simulink library "filters"  (R2024b)
settings: Solver=VariableStepAuto  StartTime=0.0  StopTime=10.0  RelTol=1e-3
libraries: simulink x1
settings Model: Creator=upattacini  LastModifiedBy=upattacini

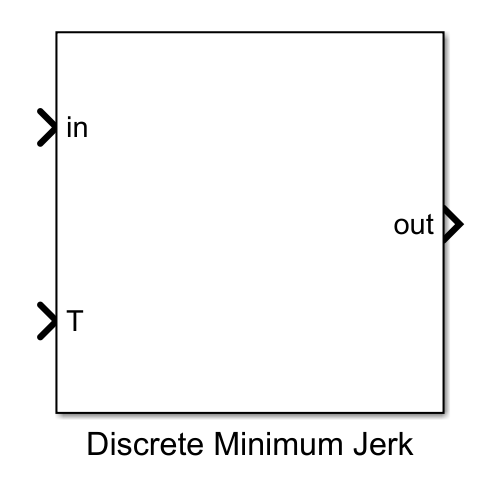
[thumbnail: Simulink's stored preview of the top-level diagram]
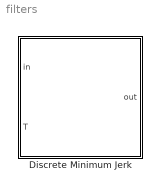
== system filters ==
  Discrete Minimum Jerk : Subsystem  mask(Minimum Jerk Filter){Ts=0.001}
      mask prompts: Ts "Sample time (s)"
      mask help:
      | Apply quasi-minimum jerk filtering to the input.
      | The filter reactivity can be adjusted via the input T, which specifies the rise-time.

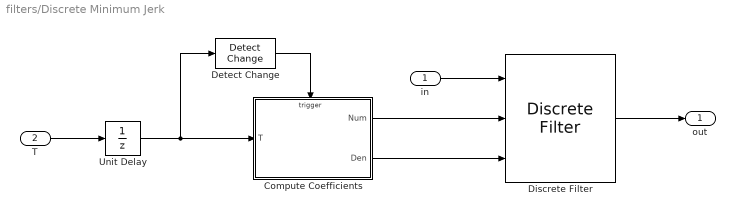
== system filters/Discrete Minimum Jerk ==
  in : Inport  PortDimensions=1
  T : Inport  Port=2  PortDimensions=1
  Compute Coefficients : Subsystem
  Detect Change : simulink/Logic and Bit Operations/Detect Change  vinit=0  OutDataTypeStr=uint8
  Discrete Filter : DiscreteFilter  NumeratorSource=Input port  DenominatorSource=Input port  a0EqualsOne=on
      settings: InputPortMap=u0,p1,p3
  Unit Delay : UnitDelay  SampleTime=Ts  HasFrameUpgradeWarning=on
  out : Outport  PortDimensions=1
  wires:
  Compute Coefficients/2(Den) -> Discrete Filter/3
  T/1 -> Unit Delay/1
  Compute Coefficients/1(Num) -> Discrete Filter/2
  Detect Change/1 -> Compute Coefficients/Trigger
  Unit Delay/1 -> Detect Change/1, Compute Coefficients/1(T)
  Discrete Filter/1 -> out/1
  in/1 -> Discrete Filter/1

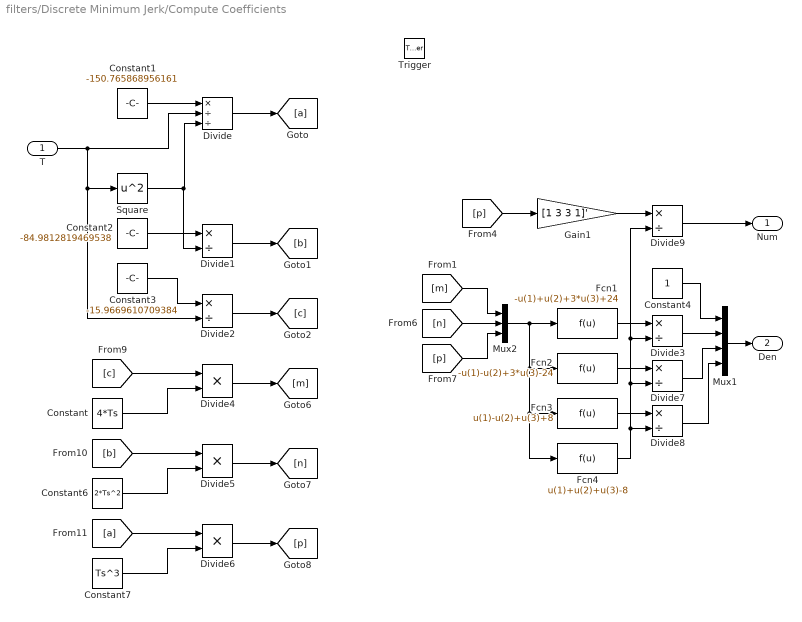
== system filters/Discrete Minimum Jerk/Compute Coefficients ==
  T : Inport
  Trigger : TriggerPort  VariantControl=(inherit)  PortDimensions=1
  Constant : Constant  Value=4*Ts
  Constant1 : Constant  Value=-150.765868956161
  Constant2 : Constant  Value=-84.9812819469538
  Constant3 : Constant  Value=-15.9669610709384
  Constant4 : Constant
  Constant6 : Constant  Value=2*Ts^2
  Constant7 : Constant  Value=Ts^3
  Divide : Product  Inputs=*//
  Divide{1..3,7..9} (6 alike) : Product  Inputs=*/
  Divide4 : Product  Inputs=**
  Divide5 : Product  Inputs=**
  Divide6 : Product  Inputs=**
  Fcn1 : Fcn  Expr=-u(1)+u(2)+3*u(3)+24
  Fcn2 : Fcn  Expr=-u(1)-u(2)+3*u(3)-24
  Fcn3 : Fcn  Expr=u(1)-u(2)+u(3)+8
  Fcn4 : Fcn  Expr=u(1)+u(2)+u(3)-8
  Gain1 : Gain  Gain=[1 3 3 1]'
  Mux1 : Mux
  Mux2 : Mux  Inputs=3
  Square : Math  Operator=square
  Num : Outport  InitialOutput=[0 0 0 0]
  Den : Outport  Port=2  InitialOutput=[1 0 0 0]'
  wires:
  Constant1/1 -> Divide/1
  Divide1/1 -> [b]
  T/1 -> Divide2/2, Square/1, Divide/2
  Divide2/1 -> [c]
  [p] -> Gain1/1
  Constant2/1 -> Divide1/1
  Constant3/1 -> Divide2/1
  Square/1 -> Divide1/2, Divide/3
  Divide/1 -> [a]
  Constant4/1 -> Mux1/1
  Mux1/1 -> Den/1
  Divide4/1 -> [m]
  [c] -> Divide4/1
  Constant/1 -> Divide4/2
  Constant6/1 -> Divide5/2
  [b] -> Divide5/1
  Divide5/1 -> [n]
  Divide6/1 -> [p]
  [a] -> Divide6/1
  Constant7/1 -> Divide6/2
  [m] -> Mux2/1
  [n] -> Mux2/2
  [p] -> Mux2/3
  Mux2/1 -> Fcn4/1, Fcn3/1, Fcn2/1, Fcn1/1
  Fcn1/1 -> Divide3/1
  Divide3/1 -> Mux1/2
  Divide7/1 -> Mux1/3
  Divide8/1 -> Mux1/4
  Fcn2/1 -> Divide7/1
  Fcn3/1 -> Divide8/1
  Fcn4/1 -> Divide8/2, Divide7/2, Divide9/2, Divide3/2
  Gain1/1 -> Divide9/1
  Divide9/1 -> Num/1
